simulink model "power_OLTCregtransformer"  (Simulink 6.0)
settings: Solver=ode23tb  StartTime=0.0  StopTime=120  MaxStep=1/60  RelTol=1e-4  AbsTol=1e-3
libraries: powerlib x75, powerlib_extras x18, simulink_extras x1
(part 1 of 3)
settings Model: Creator=batserve  LastModifiedBy=batserve  ExtModeAutoUpdateStatusClock=off
settings DataIOCC: SignalLoggingName=sigsOut
settings DebuggingCC: CheckExecutionContextPreStartOutputMsg=on  CheckExecutionContextRuntimeOutputMsg=on  SolverPrmCheckMsg=none
settings HardwareCC: TargetUnknown=on
settings ModelReferenceCC: UpdateModelReferenceTargets=IfOutOfDate

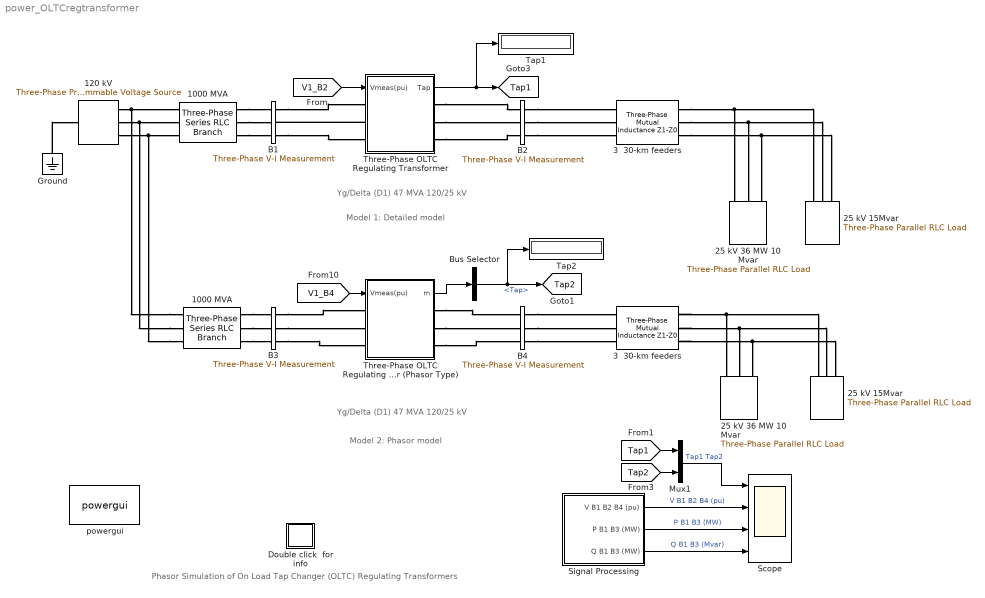
== system power_OLTCregtransformer ==
  note: Phasor Simulation of On Load Tap Changer (OLTC) Regulating Transformers
  note: Model 1: Detailed model
  note: Model 2: Phasor model
  note: Yg/Delta (D1)
      | 47 MVA 120/25 kV
  note: Yg/Delta (D1)
      | 47 MVA 120/25 kV
  1000 MVA : powerlib/Elements/Three-Phase Series RLC Branch  PhysicalDomain=powersysdomain  SubClassName=unknown  LeftPortType=p1  RightPortType=p1  LConnTagsString=A|B|C  RConnTagsString=A|B|C  Resistance=120e3^2/1000e6/10  Inductance=120e3^2/1000e6/(2*pi*60)  Capacitance=inf  Measurements=None
  "1000 MVA " : powerlib/Elements/Three-Phase Series RLC Branch  PhysicalDomain=powersysdomain  SubClassName=unknown  LeftPortType=p1  RightPortType=p1  LConnTagsString=A|B|C  RConnTagsString=A|B|C  Resistance=120e3^2/1000e6/10  Inductance=120e3^2/1000e6/(2*pi*60)  Capacitance=inf  Measurements=None
  120 kV : powerlib/Electrical Sources/Three-Phase Programmable Voltage Source  PositiveSequence=[120e3 0 60]  VariationEntity=Amplitude  VariationType=Table of time-amplitude pairs  VariationStep=0.2  VariationRate=10  VariationMagnitude=0.3  VariationFrequency=2  VariationTiming="[5  20]"  VariationPhaseA=off  Amplitudes="[ 1 0.95   1.1 ]"  TimeValues="[0  10 50]"  HarmonicGeneration=off  HarmonicA=[3 0.2 -25 0]  HarmonicB=[2 0.15 35 2]  Timing="[0.05  3]"
  25 kV 15Mvar : powerlib/Elements/Three-Phase Parallel RLC Load  Orientation=down  PhysicalDomain=powersysdomain  SubClassName=unknown  LeftPortType=p1  RightPortType=p1  LConnTagsString=A|B|C  Configuration=Y (grounded)  NominalVoltage=25e3  NominalFrequency=60  ActivePower=0  InductivePower=0  CapacitivePower=15e6  Measurements=None
  "25 kV 15Mvar " : powerlib/Elements/Three-Phase Parallel RLC Load  Orientation=down  PhysicalDomain=powersysdomain  SubClassName=unknown  LeftPortType=p1  RightPortType=p1  LConnTagsString=A|B|C  Configuration=Y (grounded)  NominalVoltage=25e3  NominalFrequency=60  ActivePower=0  InductivePower=0  CapacitivePower=15e6  Measurements=None
  25 kV 36 MW 10 Mvar : powerlib/Elements/Three-Phase Parallel RLC Load  Orientation=down  PhysicalDomain=powersysdomain  SubClassName=unknown  LeftPortType=p1  RightPortType=p1  LConnTagsString=A|B|C  Configuration=Y (grounded)  NominalVoltage=25e3  NominalFrequency=60  ActivePower=36e6  InductivePower=10e6  CapacitivePower=0  Measurements=None
  "25 kV 36 MW 10 Mvar " : powerlib/Elements/Three-Phase Parallel RLC Load  Orientation=down  PhysicalDomain=powersysdomain  SubClassName=unknown  LeftPortType=p1  RightPortType=p1  LConnTagsString=A|B|C  Configuration=Y (grounded)  NominalVoltage=25e3  NominalFrequency=60  ActivePower=36e6  InductivePower=10e6  CapacitivePower=0  Measurements=None
  3  30-km feeders : powerlib/Elements/Three-Phase Mutual Inductance Z1-Z0  PhysicalDomain=powersysdomain  SubClassName=unknown  LeftPortType=p1  RightPortType=p1  LConnTagsString=a|b|c  RConnTagsString=A|B|C  PositiveSequence=[ 0.1153 , 1.048e-3 ]*30/3  ZeroSequence=[ 0.4130 , 3.321e-3 ]*30/3
  "3  30-km feeders " : powerlib/Elements/Three-Phase Mutual Inductance Z1-Z0  PhysicalDomain=powersysdomain  SubClassName=unknown  LeftPortType=p1  RightPortType=p1  LConnTagsString=a|b|c  RConnTagsString=A|B|C  PositiveSequence=[ 0.1153 , 1.048e-3 ]*30/3  ZeroSequence=[ 0.4130 , 3.321e-3 ]*30/3
  B1 : powerlib/Measurements/Three-Phase V-I Measurement  VoltageMeasurement=phase-to-ground  SetLabelV=on  LabelV=VabcB1  Vpu=on  Vbase=120e3  CurrentMeasurement=yes  SetLabelI=on  LabelI=IabcB1  Ipu=on  Pbase=47e6  OutputType=Complex  PhasorSimulation=on  PSBequivalent=0
  B2 : powerlib/Measurements/Three-Phase V-I Measurement  VoltageMeasurement=phase-to-ground  SetLabelV=on  LabelV=VabcB2  Vpu=on  Vbase=25e3  CurrentMeasurement=no  SetLabelI=on  LabelI=IabcB2  Ipu=on  Pbase=47e6  OutputType=Complex  PhasorSimulation=on  PSBequivalent=0
  B3 : powerlib/Measurements/Three-Phase V-I Measurement  VoltageMeasurement=phase-to-ground  SetLabelV=on  LabelV=VabcB3  Vpu=on  Vbase=120e3  CurrentMeasurement=yes  SetLabelI=on  LabelI=IabcB3  Ipu=on  Pbase=47e6  OutputType=Complex  PhasorSimulation=on  PSBequivalent=0
  B4 : powerlib/Measurements/Three-Phase V-I Measurement  VoltageMeasurement=phase-to-ground  SetLabelV=on  LabelV=VabcB4  Vpu=on  Vbase=25e3  CurrentMeasurement=no  SetLabelI=on  LabelI=IabcB4  Ipu=on  Pbase=47e6  OutputType=Complex  PhasorSimulation=on  PSBequivalent=0
  Bus Selector : BusSelector  DialogController=Simulink.DDGSource_Bus  OutputSignals=Tap
  Double click  for info : Subsystem
      mask Display: disp('?')
  Ground : powerlib/Elements/Ground  Orientation=down  PhysicalDomain=powersysdomain  SubClassName=unknown  LeftPortType=p1  RightPortType=p1  LConnTagsString=a
  Mux1 : Mux  Inputs=2
  Scope : Scope  NumInputPorts=4
      settings: TimeRange=120  YMin=-8~0.9~30~5  YMax=5~1.25~50~15
  Signal Processing : Subsystem
  Tap1 : Display
      settings: SampleTime=0.1
  Tap2 : Display
      settings: SampleTime=0.1
  Three-Phase OLTC Regulating Transformer : Subsystem  mask(Three-Phase OLTC Regulating Transformer Yg/(D1) -17 positions ){ShowParam=Transformer parameters, NominalParameters=[47e6  60], Winding1=[120e3  0.003 0.09], Winding2=[25e3   0.003 0.09], RXpuTaps=[ 0.003 0.09], RXmag=[300 300], SetSaturation=off, SaturationCurrentFlux=[0 0; 0.002 1.0; 0.006 1.12; 0.009 1.15; 0.015 1.17; 0.03 1.19; 0.05 1.20; 0.08 1.21; 1.0 1.302], DeltaU=0.01875, InitialTap=-4, TapSelectionTime=4, TransferTime=0.06, Rtransfer=5, RegulatorOn=on, Regulator=[1.04  0.0375  1.0 ]}
      mask prompts: ShowParam "Show"; NominalParameters "Nominal power and frequency [ Pnom(VA)  Fnom(Hz)]:"; Winding1 "Winding 1 (Yg) [V2(Vrms Ph Ph) R1(pu)  X1(pu) ]:"; Winding2 "Winding 2 (D1) [V2(Vrms Ph Ph) R2(pu)  X2(pu) ]"; RXpuTaps "Tapped regulation winding [Rt(pu)  Xt(pu)]"; RXmag "Magnetization branch  [Rm(pu) Lm(pu)]"; SetSaturation "Simulate saturation:"; SaturationCurrentFlux "Saturation characteristic [i1 phi; i2 phi2; ....] (pu)"; DeltaU "Voltage step DeltaU per tap (pu)"; InitialTap "Initial tap position"; TapSelectionTime "Tap selection time (s) (typical 3-10s)"; TransferTime "Tap transition time (s) (typical 40-60 ms)"; Rtransfer "Transfer resistances  (ohms)"; RegulatorOn "Voltage regulator"; Regulator "Voltage regulator [ Vref(pu) DeadBand(pu)  Delay(s)]"
      mask help:
      | The On Load Tap Changer (OLTC) uses a tapped winding (regulation winding) in series with winding 1(Yg) to vary the U1 voltage in 16 DeltaU steps from tap -8 to +8 (17 positions). Tap position 0 corresponds to nominal voltage ratio.
      | The transformer voltage ratio U2/U1 (in pu) is given by:
      |                 U2/U1= 1/ (1+TapPosition*DeltaU)
      | where:
      |               -8<=TapPosition<=+8
      | In automatic mode, (Voltage regulator 'on'), the voltage regulator asks for a tap change if:
      |                  abs(Vmeas-Vref)>DeadBand/2  during a time  t > Delay.
      mask init:
      | % Below is the only line to modify
      | % to change number of taps
      | NumberOfTaps=8; 
      | 
      | if ~(abs(InitialTap)<=NumberOfTaps & (ceil(InitialTap)-InitialTap)==0)
      |    h=errordlg(sprintf('The initial tap number must be an integer comprised between % d and %d',-NumberOfTaps,NumberOfTaps),'Parameter error');
      |    uiwait(h);
      | end
      | 
      | Pnom=NominalParameters(1)/3;
      | Fnom=NominalParameters(2);
      | Vnom1= Winding1(1)/sqrt(3);
      | Vnom2=Winding2(1);
      | VnomTaps=Vnom1*DeltaU*NumberOfTaps;
      | Rpu1= Winding1(2);
      | Rpu2=Winding2(2);
      | RpuTaps=RXpuTaps(1);
      | Xpu1= Winding1(3);
      | Xpu2=Winding2(3);
      | XpuTaps=RXpuTaps(2);
      | Rm=RXmag(1);
      | Lm=RXmag(2);
      | 
      | % Saturation
      | if SetSaturation==1
      | 	set_param([gcb,'/TransformerA'],'SetSaturation','on');
      |     set_param([gcb,'/TransformerB'],'SetSaturation','on');
      |     set_param([gcb,'/TransformerC'],'SetSaturation','on');
      | else
      | 	set_param([gcb,'/TransformerA'],'SetSaturation','off');
      |     set_param([gcb,'/TransformerB'],'SetSaturation','off');
      |     set_param([gcb,'/TransformerC'],'SetSaturation','off');
      | end
      | RegulatorVref=Regulator(1);
      | RegulatorDeadBand=Regulator(2);
      | RegulatorDelay=Regulator(3);
      mask StyleString: popup(Transformer parameters|OLTC and Voltage Regulator parameters),edit,edit,edit,edit,edit,checkbox,edit,edit,edit,edit,edit,edit,popup(off|on),edit
      mask CallbackString:
      | tempMaskVis=get_param(gcb,'MaskVisibilities');
      | if strcmp(get_param(gcb,'ShowParam'),'Transformer parameters')
      | 	tempMaskVis{2}='on'; tempMaskVis{3}='on'; tempMaskVis{4}='on'; tempMaskVis{5}='on';
      | 	tempMaskVis{6}='on'; tempMaskVis{7}='on';
      | 	if strcmp(get_param(gcb,'SetSaturation'),'on')
      | 		tempMaskVis{8}='on';
      | 	end
      | 	tempMaskVis{9}='off'; tempMaskVis{10}='off'; tempMaskVis{11}='off'; tempMaskVis{12}='off';
      | 	tempMaskVis{13}='off'; tempMaskVis{14}='off'; tempMaskVis{15}='off';
      | 	set_param(gcb,'MaskVisibilities',tempMaskVis);
      | else
      | 	tempMaskVis{2}='off'; tempMaskVis{3}='off'; tempMaskVis{4}='off'; tempMaskVis{5}='off';
      | 	tempMaskVis{6}='off'; tempMaskVis{7}='off'; tempMaskVis{8}='off';
      | 	tempMaskVis{9}='on'; tempMaskVis{10}='on'; tempMaskVis{11}='on'; tempMaskVis{12}='on';
      | 	tempMaskVis{13}='on'; tempMaskVis{14}='on';
      | 	if strcmp(get_param(gcb,'RegulatorOn'),'on')
      | 		tempMaskVis{15}='on';
      | 	end
      | 	set_param(gcb,'MaskVisibilities',tempMaskVis);
      | end||||||tempMaskVis=get_param(gcb,'MaskVisibilities');
      | if strcmp(get_param(gcb,'SetSaturation'),'on') & strcmp(get_param(gcb,'ShowParam'),'Transformer parameters')
      | 	tempMaskVis{8}='on';
      | 	set_param(gcb,'MaskVisibilities',tempMaskVis);
      | else
      | 	tempMaskVis{8}='off';
      | 	set_param(gcb,'MaskVisibilities',tempMaskVis);
      | end|||||||tempMaskVis=get_param(gcb,'MaskVisibilities');
      | if strcmp(get_param(gcb,'RegulatorOn'),'on') & ~strcmp(get_param(gcb,'ShowParam'),'Transformer parameters')
      | 	tempMaskVis{15}='on';
      | 	set_param(gcb,'MaskVisibilities',tempMaskVis);
      | else
      | 	tempMaskVis{15}='off';
      | 	set_param(gcb,'MaskVisibilities',tempMaskVis);
      | end|
  Three-Phase OLTC Regulating Transformer (Phasor Type) : Subsystem  mask(Three-Phase OLTC Regulating Transformer (Phasor Type)){ShowParam=OLTC and Voltage Regulator parameters, PnomFnom=[47e6  60], Winding1=[120e3  0.003 0.09 ], Winding1Connection=Yg, Winding2=[25e3   0.003 0.09 ], Winding2Connection=Delta (D1), WindingTap=[ 0.003 0.09], RmXm=[300 300], TapOnWinding=Winding 1, dU=0.01875, TapMinMax=[ -8  +8], InitialTap=-4, TapSelectionTime=4, RegulatorOn=on, Regulator=[1.04   0.0375 1], Iw2_init=[0.7568   -45  ]}
      mask prompts: ShowParam "Show"; PnomFnom "Nominal power and frequency [Pnom (VA) Fnom(Hz)]"; Winding1 "Winding 1 [V1(Vrms Ph Ph)  R1(pu)  X1(pu)]"; Winding1Connection "Winding 1 connection"; Winding2 "Winding 2 [V2(Vrms Ph Ph)  R2(pu)  X2(pu)]"; Winding2Connection "Winding 2 connection"; WindingTap "Tapped regulation winding [Rt(pu)  Xt(pu)]"; RmXm "Magnetization branch [Rm(pu)  Xm(pu)]"; TapOnWinding "OLTC on:"; dU "Voltage step DeltaU per tap (pu)"; TapMinMax "OLTC minimum and maximum tap positions [Min Max]"; InitialTap "Initial tap position"; TapSelectionTime "Tap selection time (s) (typical 3-10s)"; RegulatorOn "Voltage regulator"; Regulator "Voltage regulator [ Vref(pu) DeadBand(pu)  Delay(s)]"; Iw2_init "Initial pos. seq. output currents of winding 2:  [Mag(pu)  Phase(deg)]"
      mask help:
      | The OLTC transformer consists of two fixed windings and a third tapped winding (regulation winding) connected in series with either winding 1 or winding 2. Voltage ratio and  transformer impedance vary with  tap position. A +30  degrees or -30 degrees phase shift  is introduced when winding 1 or winding 2 are connected in Delta.
      | In automatic mode, (Voltage regulator 'on'), the voltage regulator asks for a tap change if:
      |                  abs(Vmeas-Vref)>DeadBand/2  during a time  t > Delay.
      mask init:
      | if ~(InitialTap>=TapMinMax(1) & InitialTap<=TapMinMax(2) &(ceil(InitialTap)-InitialTap)==0)
      |    h=errordlg(sprintf('The initial tap number must be an integer comprised between % d and %d',TapMinMax(1),TapMinMax(2)),'Parameter error');
      |    uiwait(h);
      | end
      | 
      | Pnom=PnomFnom(1);
      | Fnom=PnomFnom(2);
      | w=2*pi*Fnom;
      | Vnom1=Winding1(1);
      | Vnom2=Winding2(1);
      | Ibase1=Pnom/Vnom1/sqrt(3)*sqrt(2);
      | Ibase2=Pnom/Vnom2/sqrt(3)*sqrt(2);
      | j=sqrt(-1);
      | a=exp(j*2*pi/3);
      | 
      | Z1pu=Winding1(2)+j*Winding1(3);
      | Z2pu=Winding2(2)+j*Winding2(3);
      | Ztpu=WindingTap(1)+j*WindingTap(2);
      | 
      | Nmax=max(abs(TapMinMax)); % maximum tap
      | 
      | % psi = Phase shift (deg) of winding2 with respect to winding1
      | psi=0;
      | % ks, kr = Factors used in abc_to_120 and 120_to_abc transfomation matrices
      | %          for sending end (winding 1)  and receiving end (winding 2) voltages and currents
      | % ks =0 if winding 1 connected in Delta--> zero-seq. voltage and cuurents forced to zero
      | % kr =0 if winding 2 connected in Delta--> zero-seq. voltage and cuurents forced to zero
      | ks=1; kr=1;
      | if strcmp(Winding1Connection,'Delta (D1)')
      | 	psi=psi+30;
      | 	ks=0;
      | elseif strcmp(Winding1Connection,'Delta (D11)')
      | 	psi=psi-30;
      | 	ks=0;
      | elseif strcmp(Winding1Connection,'Y')
      | 	ks=0;
      | 	kr=0;
      | end
      | if strcmp(Winding2Connection,'Delta (D1)')
      | 	psi=psi-30;
      | 	kr=0;
      | elseif strcmp(Winding2Connection,'Delta (D11)')
      | 	psi=psi+30;
      | 	kr=0;
      | elseif strcmp(Winding2Connection,'Y')
      | 	ks=0;
      | 	kr=0;
      | end
      | 
      | RegulatorVref=Regulator(1);
      | RegulatorDeadBand=Regulator(2);
      | RegulatorDelay=Regulator(3);
      | 
      | Iw2_init_mag=Iw2_init(1); % Mag pos. seq. (pu)
      | Iw2_init_pha=Iw2_init(2); % Phase pos. seq. (deg)
      | Iw2A_init_mag=Iw2_init_mag*Ibase2;
      | Iw2B_init_mag=Iw2_init_mag*Ibase2;
      | Iw2C_init_mag=Iw2_init_mag*Ibase2;
      | Iw2A_init_pha=Iw2_init_pha;
      | Iw2B_init_pha=Iw2_init_pha-120;
      | Iw2C_init_pha=Iw2_init_pha+120;
      | 
      | if TapOnWinding==1
      | 	N2_N1=1/(1+InitialTap*dU); % ratio N2/N1 tap on winding1
      | else
      | 	N2_N1=1+InitialTap*dU; %  ratio N2/N1 tap on winding2
      | end
      | 
      | Iw1A_init_mag=Iw2A_init_mag*N2_N1*Vnom2/Vnom1;
      | Iw1B_init_mag=Iw2B_init_mag*N2_N1*Vnom2/Vnom1;
      | Iw1C_init_mag=Iw2C_init_mag*N2_N1*Vnom2/Vnom1;
      | Iw1A_init_pha=Iw2A_init_pha-psi;
      | Iw1B_init_pha=Iw2B_init_pha-psi;
      | Iw1C_init_pha=Iw2C_init_pha-psi;
      | 
      | %Initialisation of pos. seq. transfer functions for breaking alg. loop
      | I21_init_real=Iw2_init_mag*cos(Iw2_init_pha*pi/180); % real pu
      | I21_init_imag=Iw2_init_mag*sin(Iw2_init_pha*pi/180); % imag pu
      mask StyleString: popup(Transformer parameters|OLTC and Voltage Regulator parameters),edit,edit,popup(Y|Yg|Delta (D1)|Delta (D11)),edit,popup(Y|Yg|Delta (D1)|Delta (D11)),edit,edit,popup(Winding 1|Winding 2),edit,edit,edit,edit,popup(off|on),edit,edit
      mask CallbackString:
      | tempMaskVis=get_param(gcb,'MaskVisibilities');
      | if strcmp(get_param(gcb,'ShowParam'),'Transformer parameters')
      | 	tempMaskVis{2}='on'; tempMaskVis{3}='on'; tempMaskVis{4}='on'; tempMaskVis{5}='on';
      | 	tempMaskVis{6}='on'; tempMaskVis{7}='on'; tempMaskVis{8}='on'; tempMaskVis{16}='on';
      | 	tempMaskVis{9}='off'; tempMaskVis{10}='off'; tempMaskVis{11}='off'; tempMaskVis{12}='off';
      | 	tempMaskVis{13}='off'; tempMaskVis{14}='off'; tempMaskVis{15}='off';
      | 	set_param(gcb,'MaskVisibilities',tempMaskVis);
      | else
      | 	tempMaskVis{2}='off'; tempMaskVis{3}='off'; tempMaskVis{4}='off'; tempMaskVis{5}='off';
      | 	tempMaskVis{6}='off'; tempMaskVis{7}='off'; tempMaskVis{8}='off'; tempMaskVis{16}='off';
      | 	tempMaskVis{9}='on'; tempMaskVis{10}='on'; tempMaskVis{11}='on'; tempMaskVis{12}='on';
      | 	tempMaskVis{13}='on'; tempMaskVis{14}='on';
      | 	if strcmp(get_param(gcb,'RegulatorOn'),'on')
      | 		tempMaskVis{15}='on';
      | 	end
      | 	set_param(gcb,'MaskVisibilities',tempMaskVis);
      | end|||||||||||||tempMaskVis=get_param(gcb,'MaskVisibilities');
      | if strcmp(get_param(gcb,'RegulatorOn'),'on') & ~strcmp(get_param(gcb,'ShowParam'),'Transformer parameters')
      | 	tempMaskVis{15}='on';
      | 	set_param(gcb,'MaskVisibilities',tempMaskVis);
      | else
      | 	tempMaskVis{15}='off';
      | 	set_param(gcb,'MaskVisibilities',tempMaskVis);
      | end||
  powergui : powerlib/powergui  Priority=2  Frange=[0:2:500]  Ylog=off  Xlog=on  save=off  variable=ZData  ZoomFFT=on  StartTime=0.0  cycles=1  DisplayStyle=1  fundamental=60  FreqAxis=off  MaxFrequency=1000  frequencyindice=1  frequencyindicesteady=1  RmsSteady=2  display=off  Ts=0  methode=on  frequency=60  echomessages=off
  tag scope: Tap1=global, Tap2=global
  wires:
  Three-Phase OLTC Regulating Transformer/1(Tap) -> [Tap1], Tap1/1
  [V1_B2] -> Three-Phase OLTC Regulating Transformer/1(Vmeas(pu))
  [V1_B4] -> Three-Phase OLTC Regulating Transformer (Phasor Type)/1(Vmeas(pu))
  Three-Phase OLTC Regulating Transformer (Phasor Type)/1(m) -> Bus Selector/1
  Bus Selector/1 -> [Tap2], Tap2/1  "<Tap>"
  [Tap1] -> Mux1/1
  [Tap2] -> Mux1/2
  Mux1/1 -> Scope/1  "Tap1 Tap2"
  Signal Processing/1(V B1 B2 B4 (pu)) -> Scope/2  "V B1 B2 B4 (pu)"
  Signal Processing/2(P B1 B3 (MW)) -> Scope/3  "P B1 B3 (MW)"
  Signal Processing/3(Q B1 B3 (MW)) -> Scope/4  "Q B1 B3 (Mvar)"
  connections:
  Three-Phase OLTC Regulating Transformer/LConn2 -- B1/RConn2
  Ground/LConn1 -- 120 kV/LConn1
  Three-Phase OLTC Regulating Transformer/RConn2 -- B2/LConn2
  Three-Phase OLTC Regulating Transformer/RConn1 -- B2/LConn1
  Three-Phase OLTC Regulating Transformer/RConn3 -- B2/LConn3
  "3  30-km feeders "/RConn1 -- 25 kV 36 MW 10 Mvar/LConn1 -- 25 kV 15Mvar/LConn1
  "3  30-km feeders "/RConn2 -- 25 kV 36 MW 10 Mvar/LConn2 -- 25 kV 15Mvar/LConn2
  "3  30-km feeders "/RConn3 -- 25 kV 36 MW 10 Mvar/LConn3 -- 25 kV 15Mvar/LConn3
  B1/RConn1 -- Three-Phase OLTC Regulating Transformer/LConn1
  B1/RConn3 -- Three-Phase OLTC Regulating Transformer/LConn3
  3  30-km feeders/RConn1 -- "25 kV 36 MW 10 Mvar "/LConn1 -- "25 kV 15Mvar "/LConn1
  3  30-km feeders/RConn2 -- "25 kV 36 MW 10 Mvar "/LConn2 -- "25 kV 15Mvar "/LConn2
  3  30-km feeders/RConn3 -- "25 kV 36 MW 10 Mvar "/LConn3 -- "25 kV 15Mvar "/LConn3
  Three-Phase OLTC Regulating Transformer (Phasor Type)/RConn1 -- B4/LConn1
  Three-Phase OLTC Regulating Transformer (Phasor Type)/RConn2 -- B4/LConn2
  Three-Phase OLTC Regulating Transformer (Phasor Type)/RConn3 -- B4/LConn3
  B3/RConn1 -- Three-Phase OLTC Regulating Transformer (Phasor Type)/LConn1
  B3/RConn2 -- Three-Phase OLTC Regulating Transformer (Phasor Type)/LConn2
  B3/RConn3 -- Three-Phase OLTC Regulating Transformer (Phasor Type)/LConn3
  1000 MVA/RConn1 -- B1/LConn1
  1000 MVA/RConn2 -- B1/LConn2
  1000 MVA/RConn3 -- B1/LConn3
  "1000 MVA "/RConn1 -- B3/LConn1
  "1000 MVA "/RConn2 -- B3/LConn2
  "1000 MVA "/RConn3 -- B3/LConn3
  "1000 MVA "/LConn1 -- 120 kV/RConn1 -- 1000 MVA/LConn1
  "1000 MVA "/LConn2 -- 120 kV/RConn2 -- 1000 MVA/LConn2
  "1000 MVA "/LConn3 -- 120 kV/RConn3 -- 1000 MVA/LConn3
  B2/RConn1 -- "3  30-km feeders "/LConn1
  B2/RConn2 -- "3  30-km feeders "/LConn2
  B2/RConn3 -- "3  30-km feeders "/LConn3
  B4/RConn1 -- 3  30-km feeders/LConn1
  B4/RConn2 -- 3  30-km feeders/LConn2
  B4/RConn3 -- 3  30-km feeders/LConn3

== system power_OLTCregtransformer/Double click  for info ==
  note: This demonstration illustrates operation of two models of On Load Tap Changer (OLTC) regulating transformer
  note: Circuit Description
  note: A   25 kV distribution network consisting of  three 30-km distribution feeders connected in parallel supplies power to a 36 MW /10 Mvar load  (0.964 PF lagging)
      | from a 120 kV, 1000 MVA system and a 120kV/25 kV OLTC regulating transformer. Reactive power compensation  is provided at load bus by a 15 Mvar capacitor bank.
      | The same circuit is duplicated in order to compare the performance of  two different models of OLTC transformers:
      |
      |     - Model 1 is a detailed model where all OLTC switches and transformer characteristics are represented. This model can be used with either continuous or discrete
      |        solvers to get detailed waveshapes or with the phasor simulation method to observe varitions of  phasor voltages and currents.
      |     - Model 2 is a simplified phasor model where the transformer and OLTC are simulated by current sources. This model can be used only with the phasor solution method
      |        It is much faster to execute and it should be the preferred model for transient stabilty studies, when several such devices are used in the same system.
      |
      | Both OLTC transformer models implement a three-phase regulating transformer rated 47 MVA, 120 kV/25 kV, Yye/ Delta, with the OLTC connected on the
      | high voltage side (120 kV). The OLTC transformers are used to regulate system voltage at 25 kV buses B2 and B4.
      |
      | Voltage regulation is performed by varying the transformer turn ratio. This is obtained by  connecting  on each phase, a tapped winding (regulation winding) in series with
      | each 120/sqrt(3)  kV winding. Nine (9) OLTC switches allow selection of 8 different taps  (tap positions 1 to 8,  plus tap 0 which provides nominal  120kV/25 kV ratio).
      | A reversing switch included in the OLTC allows reversing connections of  the regulation winding so that it  is connected either additive (positive tap positions)
      | or substractive (negative tap positions). For a  fixed 25 kV secondary voltage, each  tap provides a voltage correction of  +/-0.01875  pu or +/-1.875% of nominal 120 kV voltage.
      | Therefore, a total of 17 tap positions, incuding tap 0,  allow a voltage variation from 0.85 pu (102 kV) to 1.15 pu (138 kV) by steps of  0.01875 pu (2.25 kV).
      |
      | The positive-sequence voltages measured at buses B2 and B4 are provided as inputs to the voltage regulators (input 'Vmeas' of the transformer blocks).
      | Open the two transformer  block menus and look at  their parameters. The voltage regulators are in service ('Voltage regulator' parameter = 'on').
      | The reference voltage is set to 1.04 pu. In order to start simulation with 25-KV voltages close to 1.04 pu at buses B2 and B4, the initial tap positions are set at -4,
      | so that the transformers are boosting the voltage by a factor 1/(1-4*0.01875)=1.081.
      |
      | The detailed model is built with a fixed number of taps (8).Note that the phasor model provides more flexbility as it allows selection of  primary and secondary winding
      | connections (wye or Delta) as well as changing the number of taps and using the OLTC either on primary or secondary side.
      |
      | You can also use 'Edit/Look under mask' to see how the transformer models are built. The detailed model is built from three Multi-Winding Transformer blocks and
      | three OLTC subsystems  which contain switches performing tap selection and reversal of the regulation winding. The tap transition is performed by temporarily
      | short-circuiting two adjacent transformer taps through resistors (5 ohm resistances and 60 ms transition time as specified in the block menu) .
      | The phasor model is built with current sources emulating the transformer impedance which depends on winding resistances, leakage reactances and tap position.
      | Both models use a voltage regulator that generates pulses at the 'Up' or 'Down' outputs and  orders a tap change either in the positive or negative direction.
      | The voltage regulation depends on  the specified deadband (DB = two times the voltage step or 0.0375 pu).  This means that the maximum  voltage error at buses B2 and B4
      | should be 0.01875 pu. As long as the maximum tap number is not reached (-8 or +8), voltage should stay in the range : ( Vref-DB/2< V<1.04+DB/2 )  = (1.021< V< 1.059).
  note: G. Sybille (Hydro-Quebec)
  note: As tap selection is a relatively slow mechanical process (4 sec per tap as specified in the 'Tap selection time' parameter of the block menus), the simulation Stop time
      | is set to 2 minutes (120 s). The Three-Phase Programmable Voltage Source is used to vary the 120 kV system voltage in order to observe the OLTC performance.
      | Initially, the source is generating its nominal voltage. Then, voltage is successively decreased (0.95 pu at t = 10 s) and increased (1.10 pu at t = 50 s).
      |
      | Start the simulation and observe OLTC operation on the Scope.
      | Trace 1 shows the tap position. Trace 2 shows a superposition of positive-sequence voltages at  120 kV bus B1 (yellow ), at 25 kV bus B2 (magenta) and bus B4 (cyan).
      | Traces 3 and 4 show the active and reactive powers measured on 120 kV side (buses B1 and B3).
      |
      | When simulation starts the OLTCs are at position -4 and the resulting voltage at bus B2 and B4 is 1.038 pu.
      | At t=10 s, the source internal voltage  is suddenly lowered  to 0.95 pu , so that the 25 kV voltages drop to 0.986 pu, outside of the permitted voltage range (1.021< V<1.059).
      | The voltage regulator then orders further voltage boosting and the OLTC stabilizes at tap=-6 (V=1.025 pu)
      | At t=50 s, the souce internal voltage is suddenly increased  to 1.10 pu , so that the 25 kV voltages now reach  to 1.19 pu. The voltage regulator then starts to decrease voltage
      | by moving taps in the upward direction and the OLTCs stabilize at tap=+1 (V=1.043 pu).
  note: Demonstration
  note: Simulation with phasor model only
  note: Note: The voltage glitches observed with the phasor model when  the source voltage is stepped down (t= 10s) and up (t=50 s) can be ignored. They are caused
      |             by the first order transfer functions (one cycle time constant) which are used inside the model to break algebraic loops.
  note: In order to appreciate the gain in simulation speed provided by the phasor model, delete the detailed transformer model and replace it with a duplicate of the phasor model.
      | Restart simulation. The model runs approximately 2.5 times faster, mainly because the OLTC switches of the detailed model are not simulated.

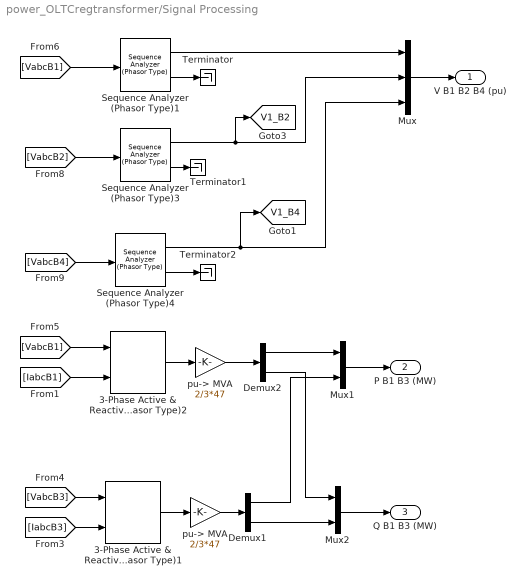
== system power_OLTCregtransformer/Signal Processing ==
  3-Phase Active & Reactive Power (Phasor Type)1 : powerlib_extras/Phasor Library/3-Phase Active & Reactive Power (Phasor Type)
  3-Phase Active & Reactive Power (Phasor Type)2 : powerlib_extras/Phasor Library/3-Phase Active & Reactive Power (Phasor Type)
  Demux1 : Demux  Outputs=2
  Demux2 : Demux  Outputs=2
  Mux : Mux  Inputs=3
  Mux1 : Mux  Inputs=2
  Mux2 : Mux  Inputs=2
  Sequence Analyzer (Phasor Type)1 : powerlib_extras/Phasor Library/Sequence Analyzer (Phasor Type)  seq=Positive
  Sequence Analyzer (Phasor Type)3 : powerlib_extras/Phasor Library/Sequence Analyzer (Phasor Type)  seq=Positive
  Sequence Analyzer (Phasor Type)4 : powerlib_extras/Phasor Library/Sequence Analyzer (Phasor Type)  seq=Positive
  Terminator : Terminator
  Terminator1 : Terminator
  Terminator2 : Terminator
  pu-> MVA : Gain  Gain=2/3*47  SaturateOnIntegerOverflow=on
  "pu-> MVA " : Gain  Gain=2/3*47  SaturateOnIntegerOverflow=on
  V B1 B2 B4 (pu) : Outport
  P B1 B3 (MW) : Outport  Port=2
  Q B1 B3 (MW) : Outport  Port=3
  tag scope: V1_B2=global, V1_B4=global
  wires:
  [VabcB1] -> Sequence Analyzer (Phasor Type)1/1
  Sequence Analyzer (Phasor Type)1/1 -> Mux/1
  [VabcB2] -> Sequence Analyzer (Phasor Type)3/1
  Sequence Analyzer (Phasor Type)3/1 -> Mux/2, [V1_B2]
  [VabcB4] -> Sequence Analyzer (Phasor Type)4/1
  Sequence Analyzer (Phasor Type)4/1 -> Mux/3, [V1_B4]
  Sequence Analyzer (Phasor Type)1/2 -> Terminator/1
  [IabcB3] -> 3-Phase Active & Reactive Power (Phasor Type)1/2
  3-Phase Active & Reactive Power (Phasor Type)1/1 -> "pu-> MVA "/1
  Demux1/1 -> Mux1/2
  Demux1/2 -> Mux2/2
  [VabcB3] -> 3-Phase Active & Reactive Power (Phasor Type)1/1
  Sequence Analyzer (Phasor Type)4/2 -> Terminator2/1
  "pu-> MVA "/1 -> Demux1/1
  Mux/1 -> V B1 B2 B4 (pu)/1
  [IabcB1] -> 3-Phase Active & Reactive Power (Phasor Type)2/2
  3-Phase Active & Reactive Power (Phasor Type)2/1 -> pu-> MVA/1
  Demux2/1 -> Mux1/1
  Demux2/2 -> Mux2/1
  pu-> MVA/1 -> Demux2/1
  [VabcB1] -> 3-Phase Active & Reactive Power (Phasor Type)2/1
  Sequence Analyzer (Phasor Type)3/2 -> Terminator1/1
  Mux1/1 -> P B1 B3 (MW)/1
  Mux2/1 -> Q B1 B3 (MW)/1

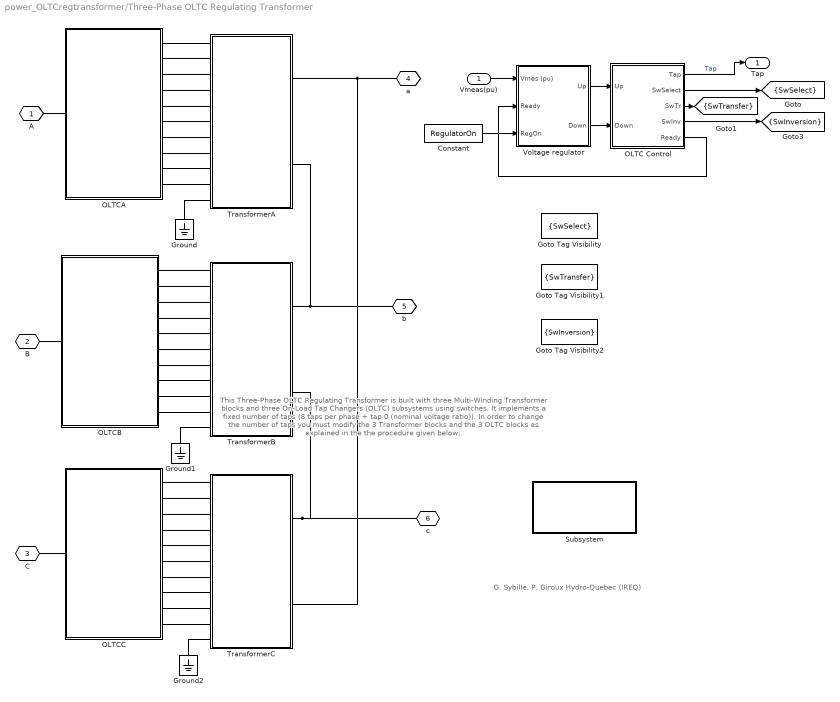
== system power_OLTCregtransformer/Three-Phase OLTC Regulating Transformer ==
  note: G. Sybille, P. Giroux Hydro-Quebec (IREQ)
  note: This Three-Phase OLTC Regulating Transformer is built with three Multi-Winding Transformer blocks
      | and three On-Load Tap Changers (OLTC) subsystems using switches.
      | It implements a fixed number of taps (8 taps per phase +  tap 0 (nominal voltage ratio)).
      |
      | In order to change the number of taps you must modify the 3 Transformer blocks
      | and the 3  OLTC blocks as explained in the  the procedure given below:
  Vmeas(pu) : Inport  Port=1  LatchInput=off
  " OLTC Control" : Subsystem  mask{NumberOfTaps=NumberOfTaps, TapSelectionTime=TapSelectionTime, TransferTime=TransferTime, InitialTap=InitialTap}
      mask prompts: NumberOfTaps "Number of taps:"; TapSelectionTime "Operating time of the tap selector (typical 3-10 s):"; TransferTime "Operating time of the transfer switch (typical 40-60 ms):"; InitialTap "Initial tap:"
      mask init:
      | TapVector=0:NumberOfTaps;
      | InitialStates=zeros(1,NumberOfTaps+1);
  Constant : Constant  Value=RegulatorOn
  Goto Tag Visibility : GotoTagVisibility  GotoTag=SwSelect
  Goto Tag Visibility1 : GotoTagVisibility  GotoTag=SwTransfer
  Goto Tag Visibility2 : GotoTagVisibility  GotoTag=SwInversion
  Ground : powerlib/Elements/Ground  Orientation=down  PhysicalDomain=powersysdomain  SubClassName=unknown  LeftPortType=p1  RightPortType=p1  LConnTagsString=a
  Ground1 : powerlib/Elements/Ground  Orientation=down  PhysicalDomain=powersysdomain  SubClassName=unknown  LeftPortType=p1  RightPortType=p1  LConnTagsString=a
  Ground2 : powerlib/Elements/Ground  Orientation=down  PhysicalDomain=powersysdomain  SubClassName=unknown  LeftPortType=p1  RightPortType=p1  LConnTagsString=a
  OLTCA : Subsystem  mask{NumberOfTaps=NumberOfTaps, InitialTap=InitialTap, Rtransfer=Rtransfer}
      mask prompts: NumberOfTaps "Nombre de prises:"; InitialTap "Prise initiale:"; Rtransfer "Resistance de court circuit (ohms):"
      mask init:
      | TapVector=0:NumberOfTaps;
      | InitialStates=zeros(1,NumberOfTaps+1);
      | InitialStates(abs(InitialTap)+1)=1;
      | 
      | InitialStateInv1=(InitialTap>=0);
      | InitialStateInv2=(InitialTap<0);
      | InitialStateInv3=InitialStateInv1;
      | InitialStateInv4=InitialStateInv2;
  OLTCB : Subsystem  mask{NumberOfTaps=NumberOfTaps, InitialTap=InitialTap, Rtransfer=Rtransfer}
      mask prompts: NumberOfTaps "Nombre de prises:"; InitialTap "Prise initiale:"; Rtransfer "Resistance de court circuit (ohms):"
      mask init: same as power_OLTCregtransformer/Three-Phase OLTC Regulating Transformer/OLTCA
  OLTCC : Subsystem  mask{NumberOfTaps=NumberOfTaps, InitialTap=InitialTap, Rtransfer=Rtransfer}
      mask prompts: NumberOfTaps "Nombre de prises:"; InitialTap "Prise initiale:"; Rtransfer "Resistance de court circuit (ohms):"
      mask init: same as power_OLTCregtransformer/Three-Phase OLTC Regulating Transformer/OLTCA
  Subsystem : Subsystem
      mask Display: disp('Procedure\n to change\n the number of taps')
  TransformerA : Subsystem  AncestorBlock=powerlib/Elements/Multi-Winding Transformer  mask(Multi-Winding Transformer){LeftWindings=2, RightWindings=1, TappedWindings=taps on upper left winding, NumberOfTaps=7, NominalPower=[Pnom  Fnom], NominalVoltages=[ VnomTaps Vnom1  Vnom2 ], WindingResistances=[ RpuTaps Rpu1 Rpu2], WindingInductances=[ XpuTaps Xpu1  Xpu2 ], SetSaturation=off, Rm=Rm, Lm=Lm, Saturation=[ 0,0 ; 0.0024,1.2 ; 1.0,1.52 ], Hysteresis=off, DataFile='hysteresis.mat', Measurements=None, InitialFlux=0, TransfoNumber=1}
      mask prompts: LeftWindings "Number of windings on left side"; RightWindings "Number of windings on right side"; TappedWindings "Tapped winding"; NumberOfTaps "----  Number of taps (equally spaced):"; NominalPower "Nominal power and frequency [Pn(VA) fn(Hz)]:"; NominalVoltages "Winding nominal voltages [U1 U2 ... Un] (Vrms):"; WindingResistances "Winding resistances [R1 R2 ... Rn] (pu):"; WindingInductances "Winding leakage inductances [L1 L2 ... Ln] (pu):"; SetSaturation "Saturable core"; Rm "Magnetization resistance  Rm (pu)"; Lm "Magnetization reactance Lm (pu)"; Saturation "Saturation characteristic (pu) [ i1 ,  phi1 ;  i2 , phi2 ; ... ]"; Hysteresis "Simulate hysteresis"; DataFile "----  Hysteresis Data Mat file"; InitialFlux "Initial Flux (internal use)"; TransfoNumber "Device number (internal use)"
      mask help:
      | Implements a transformer with multiple windings. The number of windings can be
      | specified for the left side and for the right side of the block.  Taps can be added
      | to the upper left winding or  to the upper right winding.
      mask init:
      | block = gcb;
      | [lx,ly,rx,ry,hlx,hly,hrx,hry] = powericon('NWindingsTransformerIcon');
      | %
      | powerbase = NominalPower(1);
      | wbase = 2*pi*NominalPower(2);
      | if TappedWindings>1
      | 	voltbase = NominalVoltages(1)/(NumberOfTaps+1);
      | else
      |     voltbase = NominalVoltages(1);
      | end
      | BaseCurrent = (powerbase/voltbase)*sqrt(2);
      | BaseFlux = (voltbase/wbase)*sqrt(2);
      | %
      | if SetSaturation
      | 	Saturation = [-Saturation(size(Saturation,1):-1:2,:) ; Saturation(2:size(Saturation,1),:)];
      |     SaturationCurrent = [Saturation(:,1)*BaseCurrent]';
      |     SaturationFlux = [Saturation(:,2)*BaseFlux]';
      | 	if Hysteresis
      |         InitialSlope = 1;
      | 	    [Tolerances,HT,UpperFlux,LowerFlux,Current] = powericon('inithysteresis',DataFile,BaseFlux,BaseCurrent);
      | 	    if HT.UnitsPopup == 2
      | 		    % The hysteresis characteristic is in S.I.
      | 		    % consequentely we do not need to convert the in/out signals
      | 		    % of the sfunction
      | 		    BaseCurrent = 1;
      | 		    BaseFlux = 1;
      | 	    end
      | 	end
      | end
      | %
      | %powericon('NWindingsTransformerCback',block,0);
      | Ts = powericon('NWindingsTransformerInit',block);
      mask Help: web(psbhelp);
      mask StyleString: edit,edit,popup(no taps|taps on upper left winding|taps on upper right winding),edit,edit,edit,edit,edit,checkbox,edit,edit,edit,checkbox,edit,popup(None|Winding voltages|Winding currents|Flux and excitation current ( Imag + IRm )|Flux and magnetization current ( Imag )|All measurements (V I Flux)),edit,edit
      mask CallbackString: powericon('NWindingsTransformerCback',gcb,0);|powericon('NWindingsTransformerCback',gcb,0);|powericon('NWindingsTransformerCback',gcb,1);|powericon('NWindingsTransformerCback',gcb,1);|||||powericon('NWindingsTransformerCback',gcb,0);||||powericon('NWindingsTransformerCback',gcb,0);||||
      mask Display:
      | plot(-300,-200,300,200,lx,ly,rx,ry)
      | 
      | plot([-10,-10],[-180,180])
      | plot([10,10],[-180,180])
      | 
      | color('white')
      | plot(hlx,hly,hrx,hry)
  TransformerB : Subsystem  AncestorBlock=powerlib/Elements/Multi-Winding Transformer  mask(Multi-Winding Transformer){LeftWindings=2, RightWindings=1, TappedWindings=taps on upper left winding, NumberOfTaps=7, NominalPower=[Pnom  Fnom], NominalVoltages=[ VnomTaps Vnom1  Vnom2 ], WindingResistances=[ RpuTaps Rpu1 Rpu2], WindingInductances=[ XpuTaps Xpu1  Xpu2 ], SetSaturation=off, Rm=Rm, Lm=Lm, Saturation=[ 0,0 ; 0.0024,1.2 ; 1.0,1.52 ], Hysteresis=off, DataFile='hysteresis.mat', Measurements=None, InitialFlux=0, TransfoNumber=1}
      mask prompts: LeftWindings "Number of windings on left side"; RightWindings "Number of windings on right side"; TappedWindings "Tapped winding"; NumberOfTaps "----  Number of taps (equally spaced):"; NominalPower "Nominal power and frequency [Pn(VA) fn(Hz)]:"; NominalVoltages "Winding nominal voltages [U1 U2 ... Un] (Vrms):"; WindingResistances "Winding resistances [R1 R2 ... Rn] (pu):"; WindingInductances "Winding leakage inductances [L1 L2 ... Ln] (pu):"; SetSaturation "Saturable core"; Rm "Magnetization resistance  Rm (pu)"; Lm "Magnetization reactance Lm (pu)"; Saturation "Saturation characteristic (pu) [ i1 ,  phi1 ;  i2 , phi2 ; ... ]"; Hysteresis "Simulate hysteresis"; DataFile "----  Hysteresis Data Mat file"; InitialFlux "Initial Flux (internal use)"; TransfoNumber "Device number (internal use)"
      mask help:
      | Implements a transformer with multiple windings. The number of windings can be
      | specified for the left side and for the right side of the block.  Taps can be added
      | to the upper left winding or  to the upper right winding.
      mask init: same as power_OLTCregtransformer/Three-Phase OLTC Regulating Transformer/TransformerA
      mask Help: web(psbhelp);
      mask StyleString: edit,edit,popup(no taps|taps on upper left winding|taps on upper right winding),edit,edit,edit,edit,edit,checkbox,edit,edit,edit,checkbox,edit,popup(None|Winding voltages|Winding currents|Flux and excitation current ( Imag + IRm )|Flux and magnetization current ( Imag )|All measurements (V I Flux)),edit,edit
      mask CallbackString: powericon('NWindingsTransformerCback',gcb,0);|powericon('NWindingsTransformerCback',gcb,0);|powericon('NWindingsTransformerCback',gcb,1);|powericon('NWindingsTransformerCback',gcb,1);|||||powericon('NWindingsTransformerCback',gcb,0);||||powericon('NWindingsTransformerCback',gcb,0);||||
      mask Display:
      | plot(-300,-200,300,200,lx,ly,rx,ry)
      | 
      | plot([-10,-10],[-180,180])
      | plot([10,10],[-180,180])
      | 
      | color('white')
      | plot(hlx,hly,hrx,hry)
  TransformerC : Subsystem  AncestorBlock=powerlib/Elements/Multi-Winding Transformer  mask(Multi-Winding Transformer){LeftWindings=2, RightWindings=1, TappedWindings=taps on upper left winding, NumberOfTaps=7, NominalPower=[Pnom  Fnom], NominalVoltages=[ VnomTaps Vnom1  Vnom2 ], WindingResistances=[ RpuTaps Rpu1 Rpu2], WindingInductances=[ XpuTaps Xpu1  Xpu2 ], SetSaturation=off, Rm=Rm, Lm=Lm, Saturation=[ 0,0 ; 0.0024,1.2 ; 1.0,1.52 ], Hysteresis=off, DataFile='hysteresis.mat', Measurements=None, InitialFlux=0, TransfoNumber=1}
      mask prompts: LeftWindings "Number of windings on left side"; RightWindings "Number of windings on right side"; TappedWindings "Tapped winding"; NumberOfTaps "----  Number of taps (equally spaced):"; NominalPower "Nominal power and frequency [Pn(VA) fn(Hz)]:"; NominalVoltages "Winding nominal voltages [U1 U2 ... Un] (Vrms):"; WindingResistances "Winding resistances [R1 R2 ... Rn] (pu):"; WindingInductances "Winding leakage inductances [L1 L2 ... Ln] (pu):"; SetSaturation "Saturable core"; Rm "Magnetization resistance  Rm (pu)"; Lm "Magnetization reactance Lm (pu)"; Saturation "Saturation characteristic (pu) [ i1 ,  phi1 ;  i2 , phi2 ; ... ]"; Hysteresis "Simulate hysteresis"; DataFile "----  Hysteresis Data Mat file"; InitialFlux "Initial Flux (internal use)"; TransfoNumber "Device number (internal use)"
      mask help:
      | Implements a transformer with multiple windings. The number of windings can be
      | specified for the left side and for the right side of the block.  Taps can be added
      | to the upper left winding or  to the upper right winding.
      mask init: same as power_OLTCregtransformer/Three-Phase OLTC Regulating Transformer/TransformerA
      mask Help: web(psbhelp);
      mask StyleString: edit,edit,popup(no taps|taps on upper left winding|taps on upper right winding),edit,edit,edit,edit,edit,checkbox,edit,edit,edit,checkbox,edit,popup(None|Winding voltages|Winding currents|Flux and excitation current ( Imag + IRm )|Flux and magnetization current ( Imag )|All measurements (V I Flux)),edit,edit
      mask CallbackString: powericon('NWindingsTransformerCback',gcb,0);|powericon('NWindingsTransformerCback',gcb,0);|powericon('NWindingsTransformerCback',gcb,1);|powericon('NWindingsTransformerCback',gcb,1);|||||powericon('NWindingsTransformerCback',gcb,0);||||powericon('NWindingsTransformerCback',gcb,0);||||
      mask Display:
      | plot(-300,-200,300,200,lx,ly,rx,ry)
      | 
      | plot([-10,-10],[-180,180])
      | plot([10,10],[-180,180])
      | 
      | color('white')
      | plot(hlx,hly,hrx,hry)
  Voltage regulator : Subsystem  mask{Vref=RegulatorVref, DeadBand=RegulatorDeadBand, TimeDelay=RegulatorDelay}
      mask prompts: Vref "Vref (pu)"; DeadBand "Deadband (pu)"; TimeDelay "Time delay (s)"
  A : PMIOPort  Tag=PMCPort  Port=1  Side=Left
  B : PMIOPort  Tag=PMCPort  Port=2  Side=Left
  C : PMIOPort  Tag=PMCPort  Port=3  Side=Left
  a : PMIOPort  Tag=PMCPort  Orientation=left  Port=4  Side=Right
  b : PMIOPort  Tag=PMCPort  Orientation=left  Port=5  Side=Right
  c : PMIOPort  Tag=PMCPort  Orientation=left  Port=6  Side=Right
  Tap : Outport
  tag scope: SwInversion=scoped, SwSelect=scoped, SwTransfer=scoped
  wires:
  Constant/1 -> Voltage regulator/3(RegOn)
  Vmeas(pu)/1 -> Voltage regulator/1(Vmes (pu))
  Voltage regulator/2(Down) -> " OLTC Control"/2(Down)
  " OLTC Control"/5(Ready) -> Voltage regulator/2(Ready)
  Voltage regulator/1(Up) -> " OLTC Control"/1(Up)
  " OLTC Control"/4(SwInv) -> [SwInversion]
  " OLTC Control"/1(Tap) -> Tap/1  "Tap"
  " OLTC Control"/2(SwSelect) -> [SwSelect]
  " OLTC Control"/3(SwTr) -> [SwTransfer]
  connections:
  Ground/LConn1 -- TransformerA/LConn11
  OLTCA/RConn10 -- TransformerA/LConn10
  OLTCA/RConn9 -- TransformerA/LConn9
  OLTCA/RConn8 -- TransformerA/LConn8
  OLTCA/RConn7 -- TransformerA/LConn7
  OLTCA/RConn6 -- TransformerA/LConn6
  OLTCA/RConn5 -- TransformerA/LConn5
  OLTCA/RConn4 -- TransformerA/LConn4
  OLTCA/RConn3 -- TransformerA/LConn3
  OLTCA/RConn2 -- TransformerA/LConn2
  OLTCA/RConn1 -- TransformerA/LConn1
  TransformerC/RConn1 -- c/RConn1 -- TransformerB/RConn2
  OLTCC/RConn10 -- TransformerC/LConn10
  OLTCC/RConn9 -- TransformerC/LConn9
  OLTCC/RConn8 -- TransformerC/LConn8
  OLTCC/RConn7 -- TransformerC/LConn7
  OLTCC/RConn6 -- TransformerC/LConn6
  OLTCC/RConn5 -- TransformerC/LConn5
  OLTCC/RConn4 -- TransformerC/LConn4
  OLTCC/RConn3 -- TransformerC/LConn3
  OLTCC/RConn2 -- TransformerC/LConn2
  Ground2/LConn1 -- TransformerC/LConn11
  OLTCC/RConn1 -- TransformerC/LConn1
  C/RConn1 -- OLTCC/LConn1
  OLTCB/RConn1 -- TransformerB/LConn1
  OLTCB/RConn2 -- TransformerB/LConn2
  OLTCB/RConn3 -- TransformerB/LConn3
  OLTCB/RConn4 -- TransformerB/LConn4
  OLTCB/RConn5 -- TransformerB/LConn5
  OLTCB/RConn6 -- TransformerB/LConn6
  OLTCB/RConn7 -- TransformerB/LConn7
  OLTCB/RConn8 -- TransformerB/LConn8
  OLTCB/RConn10 -- TransformerB/LConn10
  OLTCB/RConn9 -- TransformerB/LConn9
  Ground1/LConn1 -- TransformerB/LConn11
  B/RConn1 -- OLTCB/LConn1
  A/RConn1 -- OLTCA/LConn1
  TransformerC/RConn2 -- a/RConn1 -- TransformerA/RConn1
  TransformerB/RConn1 -- b/RConn1 -- TransformerA/RConn2

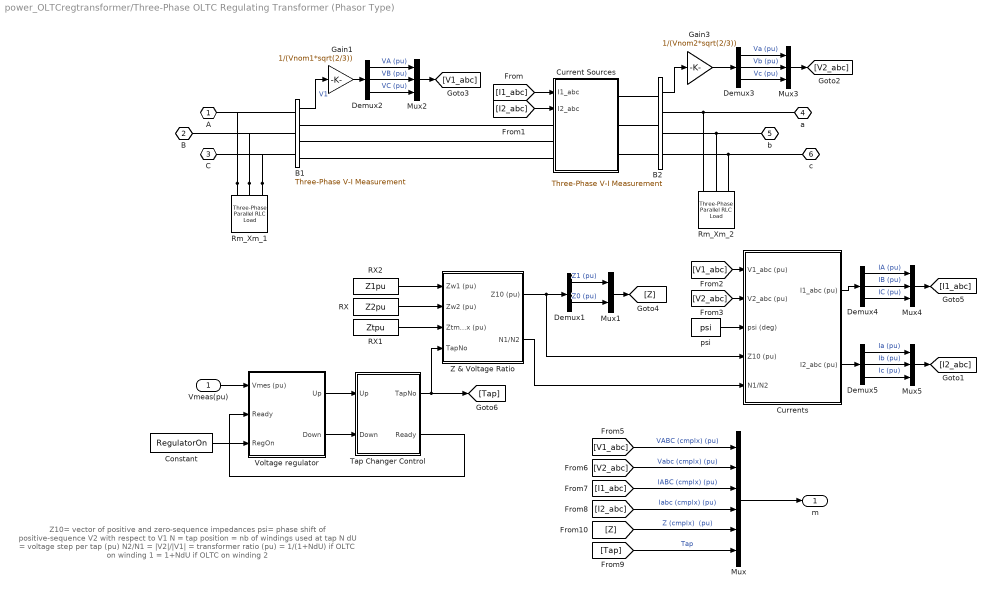
== system power_OLTCregtransformer/Three-Phase OLTC Regulating Transformer (Phasor Type) ==
  note: Z10= vector of positive and zero-sequence impedances
      | psi= phase shift of positive-sequence V2 with respect to V1
      | N =  tap position = nb of windings used at tap N
      | dU = voltage step  per tap (pu)
      | N2/N1 =  |V2|/|V1| = transformer ratio  (pu)
      |             = 1/(1+NdU)  if OLTC on winding 1
      |             = 1+NdU        if OLTC on winding 2
  Vmeas(pu) : Inport  Port=1  LatchInput=off
  " Currents " : Subsystem
  "B1 " : powerlib/Measurements/Three-Phase V-I Measurement  VoltageMeasurement=phase-to-ground  SetLabelV=off  LabelV=Vabc_B21  Vpu=off  Vbase=25e3  CurrentMeasurement=no  SetLabelI=off  LabelI=Iabc_B21  Ipu=off  Pbase=10e6  OutputType=Complex  PhasorSimulation=on  PSBequivalent=0
  B2 : powerlib/Measurements/Three-Phase V-I Measurement  VoltageMeasurement=phase-to-ground  SetLabelV=off  LabelV=Vabc_B21  Vpu=off  Vbase=25e3  CurrentMeasurement=no  SetLabelI=off  LabelI=Iabc_B21  Ipu=off  Pbase=10e6  OutputType=Complex  PhasorSimulation=on  PSBequivalent=0
  Constant : Constant  Value=RegulatorOn
  Current Sources : Subsystem
  Demux1 : Demux  Outputs=2
  Demux{2..5} (4 alike) : Demux  Outputs=3
  Gain1 : Gain  Gain=1/(Vnom1*sqrt(2/3))  SaturateOnIntegerOverflow=on
  Gain3 : Gain  Gain=1/(Vnom2*sqrt(2/3))  SaturateOnIntegerOverflow=on
  Mux : Mux  Inputs=6
  Mux1 : Mux  Inputs=2
  Mux{2..5} (4 alike) : Mux  Inputs=3
  RX : Constant  Value=Z2pu
  RX1 : Constant  Value=Ztpu
  RX2 : Constant  Value=Z1pu
  Rm_Xm_1 : powerlib/Elements/Three-Phase Parallel RLC Load  Orientation=down  PhysicalDomain=powersysdomain  SubClassName=unknown  LeftPortType=p1  RightPortType=p1  LConnTagsString=A|B|C  Configuration=Y (grounded)  NominalVoltage=Vnom1  NominalFrequency=Fnom  ActivePower=Pnom/RmXm(1)/2  InductivePower=Pnom/RmXm(2)/2  CapacitivePower=0  Measurements=None
  Rm_Xm_2 : powerlib/Elements/Three-Phase Parallel RLC Load  Orientation=down  PhysicalDomain=powersysdomain  SubClassName=unknown  LeftPortType=p1  RightPortType=p1  LConnTagsString=A|B|C  Configuration=Y (grounded)  NominalVoltage=Vnom2  NominalFrequency=Fnom  ActivePower=Pnom/RmXm(1)/2  InductivePower=Pnom/RmXm(2)/2  CapacitivePower=0  Measurements=None
  Tap Changer Control : Subsystem  mask(Tap Changer Control){MinMaxTap=TapMinMax, InitialPosition=InitialTap, MecDelay=TapSelectionTime}
      mask prompts: MinMaxTap "Minimum and maximum tap number [ Min  Max ] :"; InitialPosition "Initial tap position"; MecDelay "Mechanical delay time"
      mask init:
      | if MecDelay<=0,
      | 	MecDelay=1/60;
      | end
  Voltage regulator : Subsystem  mask{Vref=RegulatorVref, DeadBand=RegulatorDeadBand, TimeDelay=RegulatorDelay}
      mask prompts: Vref "Vref (pu)"; DeadBand "Deadband (pu)"; TimeDelay "Time delay (s)"
  Z & Voltage Ratio : Subsystem
  psi : Constant  Value=psi
  A : PMIOPort  Tag=PMCPort  Port=1  Side=Left
  B : PMIOPort  Tag=PMCPort  Port=2  Side=Left
  C : PMIOPort  Tag=PMCPort  Port=3  Side=Left
  a : PMIOPort  Tag=PMCPort  Orientation=left  Port=4  Side=Right
  b : PMIOPort  Tag=PMCPort  Orientation=left  Port=5  Side=Right
  c : PMIOPort  Tag=PMCPort  Orientation=left  Port=6  Side=Right
  m : Outport
  wires:
  " Currents "/2("I2_abc (pu) ") -> Demux5/1
  Mux5/1 -> [I2_abc]
  Demux5/3 -> Mux5/3  "Ic (pu)"
  Demux5/2 -> Mux5/2  "Ib (pu)"
  Demux5/1 -> Mux5/1  "Ia (pu)"
  " Currents "/1(I1_abc (pu)) -> Demux4/1
  Mux4/1 -> [I1_abc]
  Demux4/3 -> Mux4/3  "IC (pu)"
  Demux4/2 -> Mux4/2  "IB (pu)"
  Demux4/1 -> Mux4/1  "IA (pu)"
  Mux3/1 -> [V2_abc]
  Demux3/3 -> Mux3/3  "Vc (pu)"
  Demux3/2 -> Mux3/2  "Vb (pu)"
  Demux3/1 -> Mux3/1  "Va (pu)"
  [V1_abc] -> Mux/1  "VABC (cmplx) (pu)"
  Mux2/1 -> [V1_abc]
  Demux2/3 -> Mux2/3  "VC (pu)"
  Demux2/2 -> Mux2/2  "VB (pu)"
  Demux2/1 -> Mux2/1  "VA (pu)"
  [Z] -> Mux/5  "Z (cmplx)  (pu)"
  Mux1/1 -> [Z]
  Demux1/2 -> Mux1/2  "Z0 (pu)"
  Demux1/1 -> Mux1/1  "Z1 (pu)"
  [Tap] -> Mux/6  "Tap"
  [I2_abc] -> Mux/4  "Iabc (cmplx) (pu)"
  [I1_abc] -> Mux/3  "IABC (cmplx) (pu)"
  Mux/1 -> m/1
  [V2_abc] -> Mux/2  "Vabc (cmplx) (pu)"
  psi/1 -> " Currents "/3(psi (deg))
  [V2_abc] -> " Currents "/2(V2_abc (pu))
  [V1_abc] -> " Currents "/1(V1_abc (pu))
  Gain1/1 -> Demux2/1
  Gain3/1 -> Demux3/1
  B2/1 -> Gain3/1
  [I2_abc] -> Current Sources/2(I2_abc)
  [I1_abc] -> Current Sources/1(I1_abc)
  Z & Voltage Ratio/2(N1/N2) -> " Currents "/5(N1/N2)
  RX2/1 -> Z & Voltage Ratio/1(Zw1 (pu))
  Z & Voltage Ratio/1("Z10 (pu) ") -> " Currents "/4(Z10 (pu)), Demux1/1
  RX1/1 -> Z & Voltage Ratio/3(Ztmax (pu))
  RX/1 -> Z & Voltage Ratio/2(Zw2 (pu))
  "B1 "/1 -> Gain1/1  "V1"
  Tap Changer Control/1(TapNo) -> [Tap], Z & Voltage Ratio/4(TapNo)
  Voltage regulator/1(Up) -> Tap Changer Control/1(Up)
  Tap Changer Control/2(Ready) -> Voltage regulator/2(Ready)
  Voltage regulator/2(Down) -> Tap Changer Control/2(Down)
  Vmeas(pu)/1 -> Voltage regulator/1(Vmes (pu))
  Constant/1 -> Voltage regulator/3(RegOn)
  connections:
  Rm_Xm_1/LConn3 -- "B1 "/LConn3 -- C/RConn1
  Rm_Xm_1/LConn2 -- "B1 "/LConn2 -- B/RConn1
  Rm_Xm_1/LConn1 -- "B1 "/LConn1 -- A/RConn1
  Current Sources/LConn1 -- "B1 "/RConn1
  "B1 "/RConn2 -- Current Sources/LConn2
  "B1 "/RConn3 -- Current Sources/LConn3
  a/RConn1 -- B2/RConn1 -- Rm_Xm_2/LConn1
  b/RConn1 -- B2/RConn2 -- Rm_Xm_2/LConn2
  c/RConn1 -- B2/RConn3 -- Rm_Xm_2/LConn3
  Current Sources/RConn1 -- B2/LConn1
  Current Sources/RConn2 -- B2/LConn2
  Current Sources/RConn3 -- B2/LConn3
